simulink model "gripper_pid_tunner"  (R2021b)
settings: Solver=FixedStepAuto  StartTime=0  StopTime=Inf  RelTol=1e-3
undefined symbols (not defined in the file): Goal
libraries: robotlib x9, simulink x3, slctrlblks x2, slpidlib x1

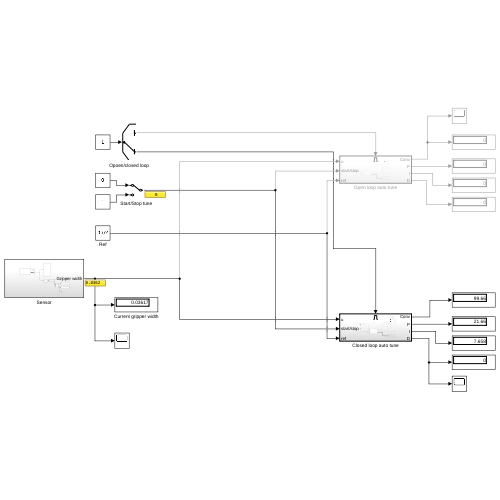
[thumbnail: Simulink's stored preview of the top-level diagram]
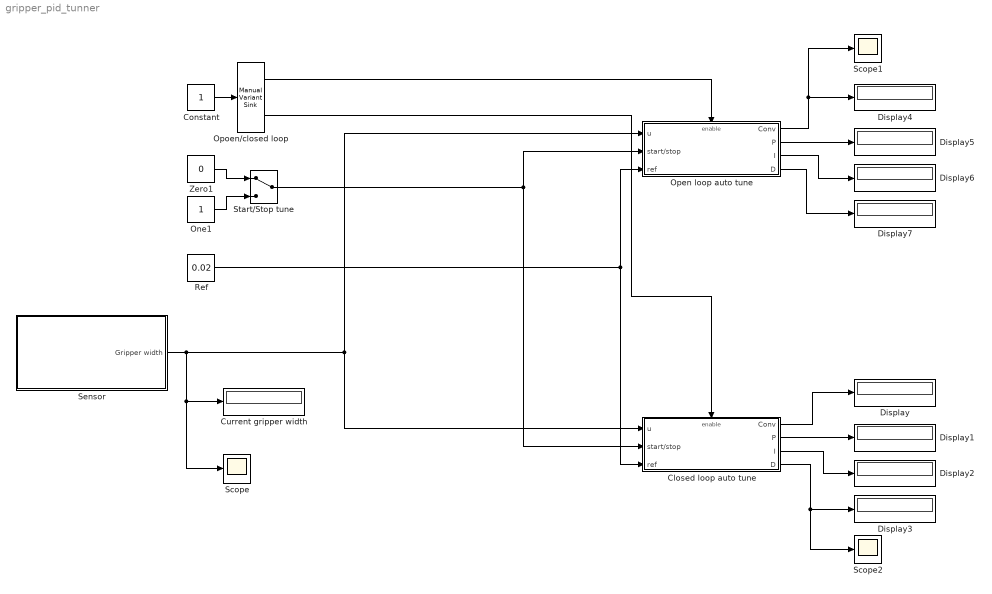
== system gripper_pid_tunner ==
  Closed loop auto tune : Subsystem
  Constant : Constant
  Current gripper width : Display
  Display{,1..7} (8 alike) : Display
  One1 : Constant  OutDataTypeStr=Inherit: Inherit via back propagation
  Open loop auto tune : Subsystem
  Opoen/closed loop : simulink/Signal Routing/Manual Variant Sink  NumChoices=2  LabelModeActiveChoice=V_2
  Ref : Constant  Value=0.02
  Scope : Scope
  Scope1 : Scope
  Scope2 : Scope
  Sensor : Subsystem
  Start/Stop tune : ManualSwitch
  Zero1 : Constant  Value=0  OutDataTypeStr=Inherit: Inherit via back propagation
  wires:
  One1/1 -> Start/Stop tune/2
  Zero1/1 -> Start/Stop tune/1
  Closed loop auto tune/1(Conv) -> Display/1
  Closed loop auto tune/2(P) -> Display1/1
  Closed loop auto tune/3(I) -> Display2/1
  Closed loop auto tune/4(D) -> Scope2/1, Display3/1
  Start/Stop tune/1 -> Closed loop auto tune/2(start/stop), Open loop auto tune/2(start/stop)
  Open loop auto tune/1(Conv) -> Scope1/1, Display4/1
  Open loop auto tune/3(I) -> Display6/1
  Open loop auto tune/4(D) -> Display7/1
  Open loop auto tune/2(P) -> Display5/1
  Ref/1 -> Closed loop auto tune/3(ref), Open loop auto tune/3(ref)
  Sensor/1(Gripper width) -> Scope/1, Current gripper width/1, Closed loop auto tune/1(u), Open loop auto tune/1(u)
  Opoen/closed loop/1 -> Open loop auto tune/Enable
  Opoen/closed loop/2 -> Closed loop auto tune/Enable
  Constant/1 -> Opoen/closed loop/1

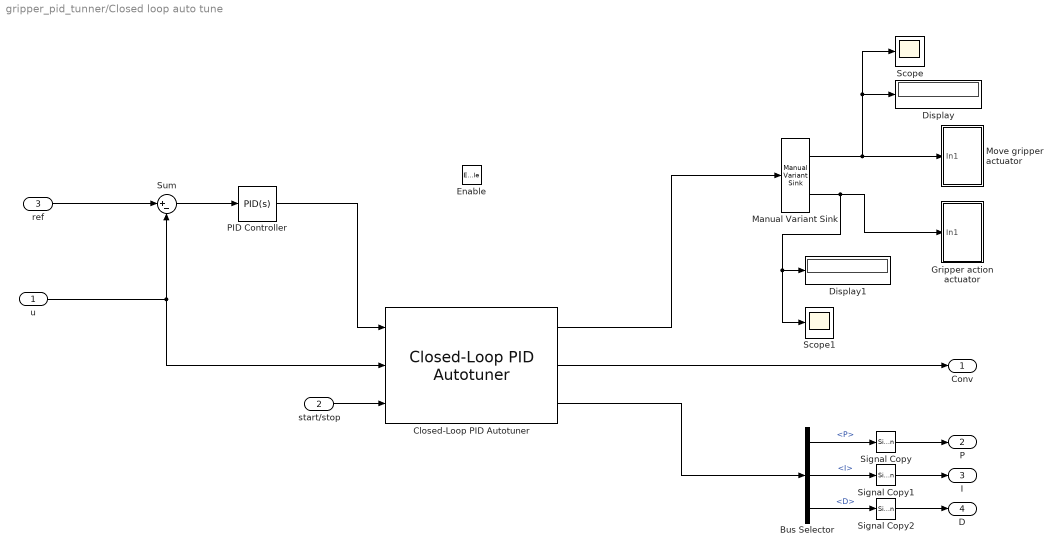
== system gripper_pid_tunner/Closed loop auto tune ==
  u : Inport
  start/stop : Inport  Port=2
  ref : Inport  Port=3
  Enable : EnablePort
  Bus Selector : BusSelector  OutputSignals=P,I,D
  Closed-Loop PID Autotuner : slctrlblks/Closed-Loop PID Autotuner  PIDType=PID  PIDForm=Parallel  TimeDomain=discrete-time  DiscreteTs=0.1  TuningTs=0.2  UseTuningTs=off  IntegratorFormula=Forward Euler  FilterFormula=Forward Euler  ContinuousTs=0.02  Bandwidth=1  UseExternalWC=off  TargetPM=60  UseExternalPM=off  UseExternalAchievedPM=off  ExperimentMode=Superposition  PlantType=Stable  PlantSign=Positive  AmpSine=0.006  UseExternalAmpSine=off  UseExternalFRD=off  UseExternalU0=off  UseCompanion=off  NotDeployTuningModule=off  UsePLCCoder=off  OutputMode=control action + perturbation  BlockDataType=double  UseConnectedPID=on  blockpath=[]  tunedP=0  tunedI=0  tunedD=0  tunedN=100  tunedPM=0  EstimationWindowSize=3  UseExternalTuningParams=off  OutputChoice=VariantCandD  SingleMultiRateVariant=SingleSamplingRate  ExperimentModeVariant=VariantSuperimposed  NumEstimationPeriods=4  NumSettlingPeriods=2
  Display : Display
  Display1 : Display
  Gripper action actuator : Subsystem
  Manual Variant Sink : simulink/Signal Routing/Manual Variant Sink  NumChoices=2  LabelModeActiveChoice=V_1
  Move gripper actuator : Subsystem
  PID Controller : slpidlib/PID Controller  Controller=PID  Form=Parallel  TimeDomain=Continuous-time  UseExternalTs=off  SampleTime=-1  IntegratorMethod=Forward Euler  FilterMethod=Forward Euler  ControllerParametersSource=internal  P=1.0  I=0  D=0  UseFilter=on  N=100  TunerSelectOption=Transfer Function Based (PID Tuner App)  InitialConditionSource=internal  InitialConditionForIntegrator=0  InitialConditionForFilter=0  DifferentiatorICPrevScaledInput=0  ExternalReset=none  TrackingMode=off  Kt=1  LimitOutput=off  SatLimitsSource=internal  UpperSaturationLimit=inf  LowerSaturationLimit=-inf  LinearizeAsGain=on  AntiWindupMode=none  Kb=1  POutMin=[]  POutMax=[]  IOutMin=[]  IOutMax=[]  DOutMin=[]  DOutMax=[]  NOutMin=[]  NOutMax=[]  SumOutMin=[]  SumOutMax=[]  SaturationOutMin=[]  SaturationOutMax=[]  PParamMin=[]  PParamMax=[]  IParamMin=[]  IParamMax=[]  DParamMin=[]  DParamMax=[]  NParamMin=[]  NParamMax=[]  KbParamMin=[]  KbParamMax=[]  KtParamMin=[]  KtParamMax=[]  KbOutMin=[]  KbOutMax=[]  KtOutMin=[]  KtOutMax=[]  IntegratorOutMin=[]  IntegratorOutMax=[]  FilterOutMin=[]  FilterOutMax=[]  SumI1OutMin=[]  SumI1OutMax=[]  SumI2OutMin=[]  SumI2OutMax=[]  SumI3OutMin=[]  SumI3OutMax=[]  SumI4OutMin=[]  SumI4OutMax=[]  SumDOutMin=[]  SumDOutMax=[]  DifferentiatorOutMin=[]  DifferentiatorOutMax=[]  FilterDiffOutCoefMin=[]  FilterDiffOutCoefMax=[]  ReciprocalOutMin=[]  ReciprocalOutMax=[]  SumDenOutMin=[]  SumDenOutMax=[]  SumNumOutMin=[]  SumNumOutMax=[]  DivideOutMin=[]  DivideOutMax=[]  UdiffTsProdOutMin=[]  UdiffTsProdOutMax=[]  NTsProdOutMin=[]  NTsProdOutMax=[]  UintegralTsProdOutMin=[]  UintegralTsProdOutMax=[]  UngainTsProdOutMin=[]  UngainTsProdOutMax=[]  IntegratorContinuousStateAttributes=''  IntegratorStateMustResolveToSignalObject=off  IntegratorRTWStateStorageClass=Auto  FilterContinuousStateAttributes=''  FilterStateMustResolveToSignalObject=off  FilterRTWStateStorageClass=Auto  ParallelPVariant=InternalParameters  IdealPVariant=Disabled  IVariant=InternalParameters  DVariant=InternalParameters  IntegratorVariant=Continuous  SatVariant=Disabled  AWVariant=Passthrough  PCopyVariant=Disabled  TRVariant=Disabled  FdbkBlocksVariant=Forward  IdealPFdbkVariant=Disabled  SatFdbkVariant=Disabled  DerivativeFilterVariant=ContFilter  NVariant=InternalParameters  NCopyVariant=Disabled  FilterICVariant=InternalICsFilter  IntegratorICVariant=InternalICs  ExternalResetVariant=Disabled  TRSumVariant=Passthrough  SumFdbkVariant=Disabled  SumVariant=Sum_PID  TsampFilterVariant=InternalTs  TsampNgainVariant=Passthrough  TsampIntegralVariant=Passthrough  ExternalSaturationOutDataTypeStr=Inherit: Same as second input
  Scope : Scope
  Scope1 : Scope
  Signal Copy : SignalConversion  OverrideOpt=off
  Signal Copy1 : SignalConversion  OverrideOpt=off
  Signal Copy2 : SignalConversion  OverrideOpt=off
  Sum : Sum  Inputs=|+-
  Conv : Outport
  P : Outport  Port=2
  I : Outport  Port=3
  D : Outport  Port=4
  wires:
  Closed-Loop PID Autotuner/3 -> Bus Selector/1
  Bus Selector/1 -> Signal Copy/1  "<P>"
  Manual Variant Sink/2 -> Scope1/1, Display1/1, Gripper action actuator/1(In1)
  Signal Copy2/1 -> D/1
  Signal Copy1/1 -> I/1
  Manual Variant Sink/1 -> Scope/1, Display/1, Move gripper actuator/1(In1)
  Bus Selector/2 -> Signal Copy1/1  "<I>"
  u/1 -> Sum/2, Closed-Loop PID Autotuner/2
  PID Controller/1 -> Closed-Loop PID Autotuner/1
  Closed-Loop PID Autotuner/2 -> Conv/1
  Bus Selector/3 -> Signal Copy2/1  "<D>"
  Signal Copy/1 -> P/1
  start/stop/1 -> Closed-Loop PID Autotuner/3
  ref/1 -> Sum/1
  Sum/1 -> PID Controller/1
  Closed-Loop PID Autotuner/1 -> Manual Variant Sink/1

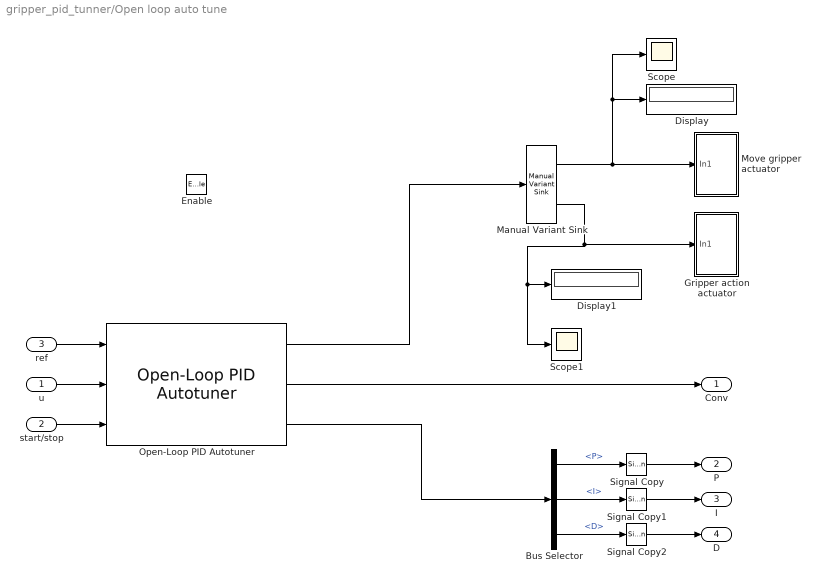
== system gripper_pid_tunner/Open loop auto tune ==
  u : Inport
  start/stop : Inport  Port=2
  ref : Inport  Port=3
  Enable : EnablePort
  Bus Selector : BusSelector  OutputSignals=P,I,D
  Display : Display
  Display1 : Display
  Gripper action actuator : Subsystem
  Manual Variant Sink : simulink/Signal Routing/Manual Variant Sink  NumChoices=2  LabelModeActiveChoice=V_2
  Move gripper actuator : Subsystem
  Open-Loop PID Autotuner : slctrlblks/Open-Loop PID Autotuner  PIDType=PID  PIDForm=Parallel  TimeDomain=discrete-time  DiscreteTs=0.1  IntegratorFormula=Forward Euler  FilterFormula=Forward Euler  ContinuousTs=0.02  Bandwidth=1  UseExternalWC=off  TargetPM=60  UseExternalPM=off  UseExternalAchievedPM=off  AmpSine=0.006  UseExternalAmpSine=off  EstimateDCGain=off  AmpStep=0.04  UseExternalAmpStep=off  UseExternalFRD=off  UseExternalU0=off  UseExternalDCGain=off  NotDeployTuningModule=off  UsePLCCoder=off  BlockDataType=double  UseConnectedPID=on  blockpath=[]  tunedP=0  tunedI=0  tunedD=0  tunedN=100  tunedPM=0  EstimationWindowSize=3
  Scope : Scope
  Scope1 : Scope
  Signal Copy : SignalConversion  OverrideOpt=off
  Signal Copy1 : SignalConversion  OverrideOpt=off
  Signal Copy2 : SignalConversion  OverrideOpt=off
  Conv : Outport
  P : Outport  Port=2
  I : Outport  Port=3
  D : Outport  Port=4
  wires:
  Open-Loop PID Autotuner/3 -> Bus Selector/1
  Bus Selector/1 -> Signal Copy/1  "<P>"
  Manual Variant Sink/2 -> Scope1/1, Display1/1, Gripper action actuator/1(In1)
  Signal Copy2/1 -> D/1
  Signal Copy1/1 -> I/1
  Manual Variant Sink/1 -> Scope/1, Display/1, Move gripper actuator/1(In1)
  Bus Selector/2 -> Signal Copy1/1  "<I>"
  u/1 -> Open-Loop PID Autotuner/2
  Open-Loop PID Autotuner/2 -> Conv/1
  Bus Selector/3 -> Signal Copy2/1  "<D>"
  Signal Copy/1 -> P/1
  start/stop/1 -> Open-Loop PID Autotuner/3
  Open-Loop PID Autotuner/1 -> Manual Variant Sink/1
  ref/1 -> Open-Loop PID Autotuner/1

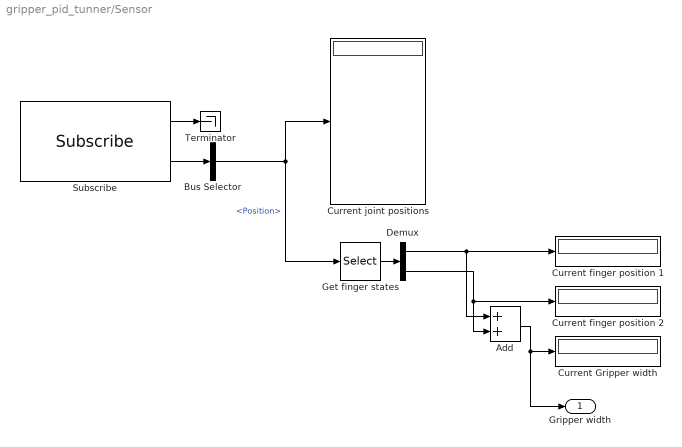
== system gripper_pid_tunner/Sensor ==
  Add : Sum
  Bus Selector : BusSelector  OutputSignals=Position
  Current Gripper width : Display
  Current finger position 1 : Display
  Current finger position 2 : Display
  Current joint positions : Display
  Demux : Demux  Outputs=2
  Get finger states : Selector  InputPortWidth=128  IndexOptions=Index vector (dialog)  Indices=[9 8]  OutputSizes=1
  Subscribe : robotlib/Subscribe  topicSource=Select from ROS network  topic=/panda/joint_states  messageType=sensor_msgs/JointState  SampleTime=-1  legacyBusStruct=off  messageQueueLength=1
  Terminator : Terminator
  Gripper width : Outport
  wires:
  Get finger states/1 -> Demux/1
  Demux/2 -> Add/2, Current finger position 2/1
  Subscribe/2 -> Bus Selector/1
  Bus Selector/1 -> Current joint positions/1, Get finger states/1  "<Position>"
  Demux/1 -> Add/1, Current finger position 1/1
  Add/1 -> Gripper width/1, Current Gripper width/1
  Subscribe/1 -> Terminator/1

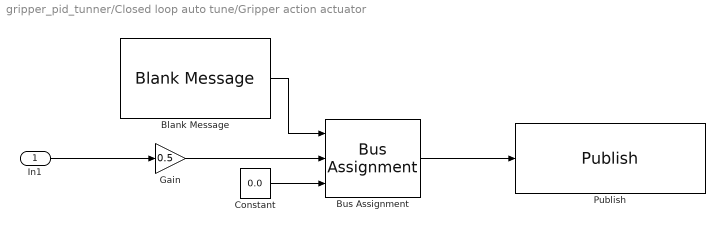
== system gripper_pid_tunner/Closed loop auto tune/Gripper action actuator ==
  In1 : Inport
  Blank Message : robotlib/Blank Message  messageClass=Message  entityType=control_msgs/GripperCommandActionGoal  messageType=control_msgs/GripperCommandActionGoal  SampleTime=inf  legacyBusStruct=off
  Bus Assignment : BusAssignment  AssignedSignals=Goal.Command.Position,Goal.Command.MaxEffort
  Constant : Constant  Value=0.0
  Gain : Gain  Gain=0.5
  Publish : robotlib/Publish  topicSource=Select from ROS network  topic=/panda/franka_gripper/gripper_action/goal  messageType=control_msgs/GripperCommandActionGoal  legacyBusStruct=off  messageQueueLength=1
  wires:
  Blank Message/1 -> Bus Assignment/1
  Constant/1 -> Bus Assignment/3
  In1/1 -> Gain/1
  Bus Assignment/1 -> Publish/1
  Gain/1 -> Bus Assignment/2

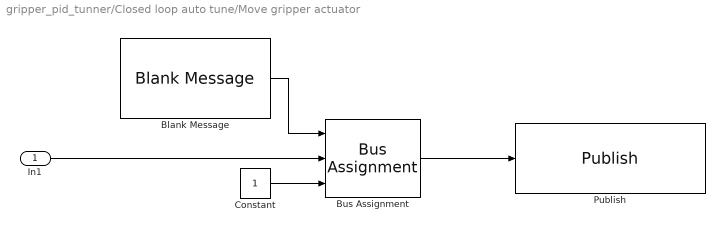
== system gripper_pid_tunner/Closed loop auto tune/Move gripper actuator ==
  In1 : Inport
  Blank Message : robotlib/Blank Message  messageClass=Message  entityType=franka_gripper/MoveActionGoal  messageType=franka_gripper/MoveActionGoal  SampleTime=inf  legacyBusStruct=off
  Bus Assignment : BusAssignment  AssignedSignals=Goal.Width,Goal.Speed
  Constant : Constant
  Publish : robotlib/Publish  topicSource=Select from ROS network  topic=/panda/franka_gripper/move/goal  messageType=franka_gripper/MoveActionGoal  legacyBusStruct=off  messageQueueLength=1
  wires:
  Blank Message/1 -> Bus Assignment/1
  Constant/1 -> Bus Assignment/3
  In1/1 -> Bus Assignment/2
  Bus Assignment/1 -> Publish/1

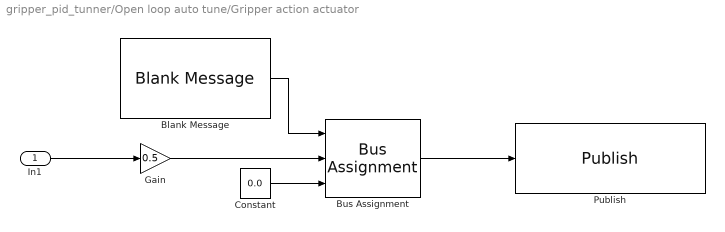
== system gripper_pid_tunner/Open loop auto tune/Gripper action actuator ==
  In1 : Inport
  Blank Message : robotlib/Blank Message  messageClass=Message  entityType=control_msgs/GripperCommandActionGoal  messageType=control_msgs/GripperCommandActionGoal  SampleTime=inf  legacyBusStruct=off
  Bus Assignment : BusAssignment  AssignedSignals=Goal.Command.Position,Goal.Command.MaxEffort
  Constant : Constant  Value=0.0
  Gain : Gain  Gain=0.5
  Publish : robotlib/Publish  topicSource=Select from ROS network  topic=/panda/franka_gripper/gripper_action/goal  messageType=control_msgs/GripperCommandActionGoal  legacyBusStruct=off  messageQueueLength=1
  wires:
  Blank Message/1 -> Bus Assignment/1
  Constant/1 -> Bus Assignment/3
  In1/1 -> Gain/1
  Bus Assignment/1 -> Publish/1
  Gain/1 -> Bus Assignment/2

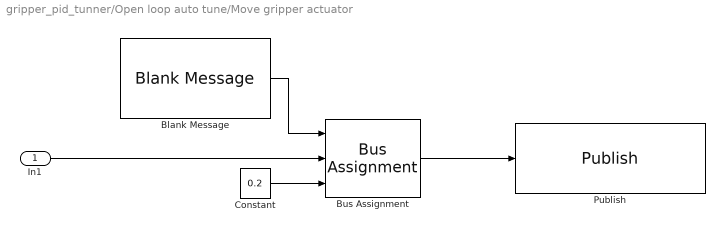
== system gripper_pid_tunner/Open loop auto tune/Move gripper actuator ==
  In1 : Inport
  Blank Message : robotlib/Blank Message  messageClass=Message  entityType=franka_gripper/MoveActionGoal  messageType=franka_gripper/MoveActionGoal  SampleTime=inf  legacyBusStruct=off
  Bus Assignment : BusAssignment  AssignedSignals=Goal.Width,Goal.Speed
  Constant : Constant  Value=0.2
  Publish : robotlib/Publish  topicSource=Select from ROS network  topic=/panda/franka_gripper/move/goal  messageType=franka_gripper/MoveActionGoal  legacyBusStruct=off  messageQueueLength=1
  wires:
  Blank Message/1 -> Bus Assignment/1
  Constant/1 -> Bus Assignment/3
  In1/1 -> Bus Assignment/2
  Bus Assignment/1 -> Publish/1
